simulink library "kpc"  (Simulink 8.1)
settings: Solver=ode1  StartTime=0.0  StopTime=Inf  FixedStep=0.001  RelTol=1e-3
PostLoadFcn:
  | , if any(exist('dsrtsu_mdlpostloadfcn', 'file') == [2, 3, 6]), try dsrtsu_mdlpostloadfcn('Execute', bdroot); catch fprintf('Error in PostLoadFcn (dsrtsu_mdlpostloadfcn) for model "%s":\n %s\n', bdroot, lasterr); end, end,
undefined symbols (not defined in the file or in its folder): AACC_VehSpdPID_kph, FALSE, KACC_ACCGapKpParamTrans_num, KACC_ACCRelSpdKpTrans_kph, KACC_ACCTGapTransMargin_s, KJUD_ACCMinTimeGap_s, MACC_TGapRefSpdKp_num, TRUE
libraries: hcu_lib x2
settings Model: DSRTSU_INTERNAL_RTI_VER=450  DSRTSU_INTERNAL_RTI_TYPE=rti1401  RTICANMMDATA=struct('GeneralSetupData',struct('modelroot','D:\ELN150201_TAIWAN\trunk\AdasDragon\software\sw_development\arch\app\acc','generalsettings',struct('filesettings',struct('destfolder',struct('Name','RTICANMM_FILES','Check',1),'buildfolder',struct('Name','.','Check',1),'AbsDestfolder',struct('Name','D:\ELN150201_TAIWAN\trunk\AdasDragon\software\sw_development\arch\app\acc\RTICANMM_FILES'),'AbsBuildfolder',struct('Name','D:\ELN150201_TAIWAN\trunk\AdasDragon\software\sw_development\arch\app\acc'))),'options',struct('addpaths',1,'rmpaths',1,'addtrcexclusion',logical(1),'cannavigator',struct('checkmonitoring',0),'show_usrtrc',0,'use_usrtrc',0),'advanced',struct('options',[1 1 1 1 1 1 1 1 1 1 1 1 1 1 1 1 1 1 1 1 1 1 1 1 1 1 1 1 1 1 1 1 1 1 1 1 1 1 1 1 1 1 1 1 1 1 1 1 1 1 1 1 1 1 1 1 1 1 1 1 1 1 1 1 1 1 1 1 1 1 1 1 1 1 1 1 1 1 1 1 1 1 1 1 1 1 1 1 1 1 1 1 1 1 1 1 1 1 1 1]),'MPSetup',{{}},'modelname','kpc','block','kpc'))  DSRTSU_INTERNAL_RTIFPGA=40  Creator=AT015555  LastModifiedBy=AT015555

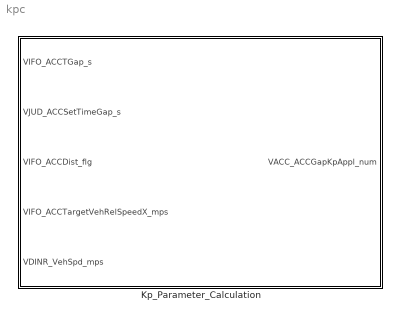
== system kpc ==
  Kp_Parameter_Calculation : Subsystem

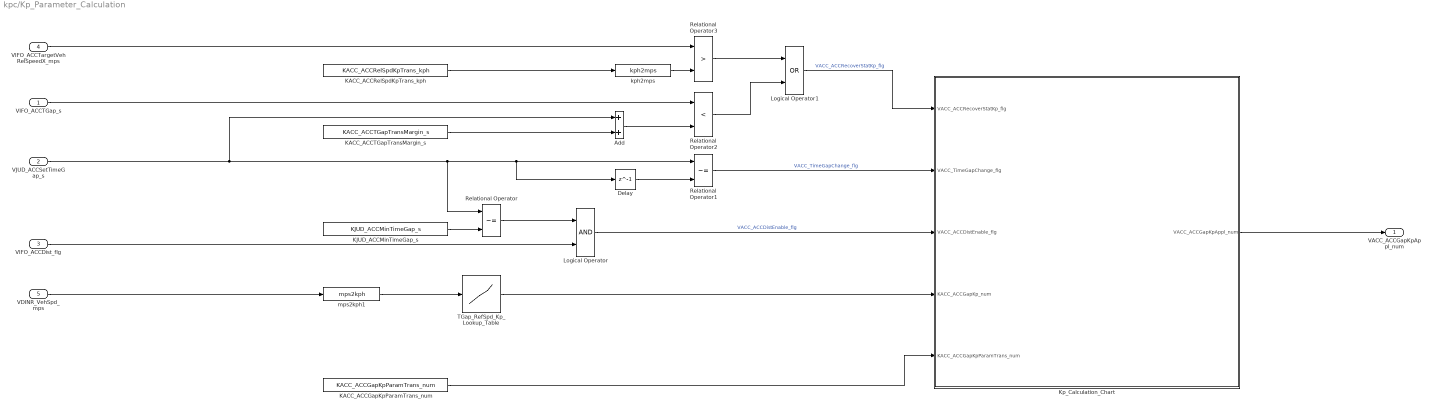
== system kpc/Kp_Parameter_Calculation ==
  VIFO_ACCTGap_s : Inport
  VJUD_ACCSetTimeGap_s : Inport  Port=2
  VIFO_ACCDist_flg : Inport  Port=3
  VIFO_ACCTargetVehRelSpeedX_mps : Inport  Port=4
  VDINR_VehSpd_mps : Inport  Port=5
  Add : Sum
  Delay : Delay  DelayLength=1  InitialCondition=0
  KACC_ACCGapKpParamTrans_num : Constant  Value=KACC_ACCGapKpParamTrans_num
  KACC_ACCRelSpdKpTrans_kph : Constant  Value=KACC_ACCRelSpdKpTrans_kph
  KACC_ACCTGapTransMargin_s : Constant  Value=KACC_ACCTGapTransMargin_s
  KJUD_ACCMinTimeGap_s : Constant  Value=KJUD_ACCMinTimeGap_s
  Kp_Calculation_Chart : Stateflow chart  TreatAsAtomicUnit=on
  Logical Operator : Logic  AllPortsSameDT=off  OutDataTypeStr=boolean
  Logical Operator1 : Logic  Operator=OR  AllPortsSameDT=off  OutDataTypeStr=boolean
  Relational Operator : RelationalOperator  Operator=~=  OutDataTypeStr=boolean
  Relational Operator1 : RelationalOperator  Operator=~=  OutDataTypeStr=boolean
  Relational Operator2 : RelationalOperator  Operator=<  OutDataTypeStr=boolean
  Relational Operator3 : RelationalOperator  Operator=>  OutDataTypeStr=boolean
  TGap_RefSpd_Kp_Lookup_Table : Lookup_n-D  NumberOfTableDimensions=1  BreakpointsForDimension1=AACC_VehSpdPID_kph  Table=MACC_TGapRefSpdKp_num  ExtrapMethod=Clip  UseLastTableValue=on  RndMeth=Simplest  InputSameDT=on
  kph2mps : hcu_lib/kph2mps
  mps2kph1 : hcu_lib/mps2kph
  VACC_ACCGapKpAppl_num : Outport
  wires:
  Logical Operator1/1 -> Kp_Calculation_Chart/1(VACC_ACCRecoverStatKp_flg)  "VACC_ACCRecoverStatKp_flg"
  KACC_ACCTGapTransMargin_s/1 -> Add/2
  Relational Operator1/1 -> Kp_Calculation_Chart/2(VACC_TimeGapChange_flg)  "VACC_TimeGapChange_flg"
  Add/1 -> Relational Operator2/2
  Relational Operator/1 -> Logical Operator/1
  Logical Operator/1 -> Kp_Calculation_Chart/3(VACC_ACCDistEnable_flg)  "VACC_ACCDistEnable_flg"
  KJUD_ACCMinTimeGap_s/1 -> Relational Operator/2
  Delay/1 -> Relational Operator1/2
  VJUD_ACCSetTimeGap_s/1 -> Relational Operator1/1, Delay/1, Relational Operator/1, Add/1
  Kp_Calculation_Chart/1(VACC_ACCGapKpAppl_num) -> VACC_ACCGapKpAppl_num/1
  VIFO_ACCTGap_s/1 -> Relational Operator2/1
  VIFO_ACCDist_flg/1 -> Logical Operator/2
  KACC_ACCGapKpParamTrans_num/1 -> Kp_Calculation_Chart/5(KACC_ACCGapKpParamTrans_num)
  KACC_ACCRelSpdKpTrans_kph/1 -> kph2mps/1
  kph2mps/1 -> Relational Operator3/2
  VIFO_ACCTargetVehRelSpeedX_mps/1 -> Relational Operator3/1
  Relational Operator3/1 -> Logical Operator1/1
  Relational Operator2/1 -> Logical Operator1/2
  TGap_RefSpd_Kp_Lookup_Table/1 -> Kp_Calculation_Chart/4(KACC_ACCGapKp_num)
  mps2kph1/1 -> TGap_RefSpd_Kp_Lookup_Table/1
  VDINR_VehSpd_mps/1 -> mps2kph1/1

== stateflow chart Kp_Parameter_Calculation/Kp_Calculation_Chart ==
  state STATIONARY
    du:
    VACC_ACCGapKpAppl_num=KACC_ACCGapKp_num;
  state FIRST_TRANSITORY
    en:
    VACC_ACCGapKpAppl_num=KACC_ACCGapKpParamTrans_num;
  state SECOND_TRANSITORY
    en:
    VACC_ACCGapKpAppl_num=KACC_ACCGapKpParamTrans_num;
  (default) -> STATIONARY
  FIRST_TRANSITORY -> SECOND_TRANSITORY : [VACC_TimeGapChange_flg==TRUE]
  STATIONARY -> FIRST_TRANSITORY : [VACC_ACCDistEnable_flg==TRUE]
  SECOND_TRANSITORY -> FIRST_TRANSITORY [order 1] : [VACC_ACCDistEnable_flg==TRUE]
  SECOND_TRANSITORY -> STATIONARY [order 2] : [VACC_ACCRecoverStatKp_flg==TRUE...
      | && VACC_ACCDistEnable_flg == FALSE ]
  data: VACC_ACCRecoverStatKp_flg input double; VACC_TimeGapChange_flg input double; VACC_ACCDistEnable_flg input double; KACC_ACCGapKp_num input double; KACC_ACCGapKpParamTrans_num input double; VACC_ACCGapKpAppl_num output single; TRUE parameter boolean; FALSE parameter boolean
